simulink model "ControlSystem_new"  (R2019a)
settings: Solver=VariableStepAuto  StartTime=0.0  StopTime=50  RelTol=1e-3
model workspace (MAT data in the model file):
  a_1 = 0
  a_2 = 0
  delta = 0.001
values from neighbouring files (symbols this model uses):
  A = [0 0 0 0 1 0 0 0 0 0 0 0 ... (64 elements, 8x8)]    [IC_4DOF_new.mat]
  a1_dim = 0.409090909091    [IC_4DOF_new.mat]
  a2_dim = 0.409090909091    [IC_4DOF_new.mat]
  Ax_dim = 0.000833333333333    [IC_4DOF_new.mat]
  delta_dim = 1    [IC_4DOF_new.mat]
  h = 0.0002    [IC_4DOF_new.mat]
  h_dim = 0.00909090909091    [IC_4DOF_new.mat]
  i0_dim = 0.0007    [IC_4DOF_new.mat]
  omega = 1047.1975512    [IC_4DOF_new.mat]
  omega_dim = 0.753327454075    [IC_4DOF_new.mat]
  P2 = 8.714    [IC_4DOF_new.mat]
  p_dim = 0    [IC_4DOF_new.mat]
  Pk = 1000000    [IC_4DOF_new.mat]
  Px_dim = 0    [IC_4DOF_new.mat]
  Sf = 1.2    [IC_4DOF_new.mat]
  Sm = 0.000315532958163    [IC_4DOF_new.mat]
  Zb = [1 0 1 0 0 1 0 1 0 0.409090909091 0 -0.409090909091 ... (16 elements, 4x4)]    [IC_4DOF_new.mat]
  Zb_1 = [0.5 0 0 -1.22222222222 0 0.5 1.22222222222 0 0.5 0 0 1.22222222222 ... (16 elements, 4x4)]    [IC_4DOF_new.mat]
libraries: simulink x25, cstblocks x1, neural x1
settings Model: Creator=Vladimir  LastModifiedBy=first
settings SolverCC: AlgebraicLoopSolver=LineSearch
settings DataIOCC: ReturnWorkspaceOutputs=off
settings DebuggingCC: ArithmeticOperatorsInVariantConditions=warning

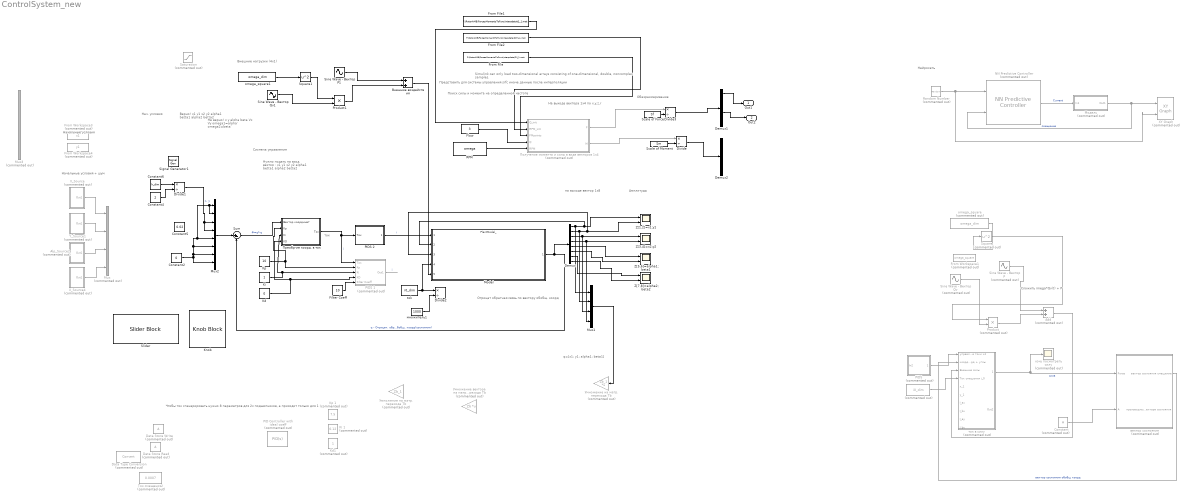
== system ControlSystem_new ==
  note: Представить для системы управления srfc иначе данные после интерполяции
  note: Simulink can only load two-dimensional arrays consisting of one-dimensional, double, noncomplex samples.
  note: Обезразмеривание
  note: На выходе вектора 1х4 по x,y,z,r
  note: Поиск силы и момента на определенной частоте
  note: Не верно!
      | x
      | y
      | alpha
      | beta
      | Vx
      | Vy
      | omega1=alpha'
      | omega2=beta'
  note: Амплитуды
  note: Система управления
  note: на выходе вектор 1x8
  note: Нужно подать на вход вектор :
      | x1
      | y1
      | x2
      | y2
      | alpha1
      | betta1
      | alpha2
      | betta2
  note: q=[x1; y1; alpha1; beta1]
  note: Нач. условия
  note: Чтобы ток сгенерировать нужно 8 параметров для 2х подшипников, а приходит только для 1
  note: Нейросеть
  note: Начальные условия
  note: Отрицат обратная связь по вектору обобщ. коорд
  note: Сложить imega*Qv(t) + P
  note: Начальные условия + шум
  note: ток
  note: Верно!
      | x1
      | y1
      | x2
      | y2
      | alpha1
      | betta1
      | alpha2
      | betta2
  note: Внешние нагрузки (4x1)
  " " : Constant  Commented=on  Value=i0_dim
  " tok" : Constant  Value=i0_dim
  " Ток смещения2" : Constant  Commented=on  Value=0.0007
  " вектор состояния " : Subsystem  Commented=on
  Add : Sum  Commented=on
  Alp_Source2 : Subsystem  Commented=on
  Constant : Constant  Commented=on  Value=A
  Constant2 : Constant  Value=0
  Constant4 : Constant  Value=2
  Constant5 : Constant  Value=0.02
  Constant6 : Constant  Value=h_dim
  Data Store Read : DataStoreRead  Commented=on
  Data Store Write : DataStoreWrite  Commented=on
  Data Type Conversion : DataTypeConversion  Commented=on
  Demux : Demux  Outputs=8
  Demux1 : Demux
  Demux2 : Demux
  Divide{,1..3} (4 alike) : Product  Inputs=*/
  "Filter Coeff " : Constant  Value=10
  "Flow " : Constant  Value=3
  From Workspace1 : FromWorkspace  Commented=on  VariableName=omega_square  SampleTime=0
  From Workspace3 : FromWorkspace  Commented=on  VariableName=x1  SampleTime=0
  From Workspace4 : FromWorkspace  Commented=on  VariableName=y1  SampleTime=0
  From File : FromFile  FileName=F:\RotorAMB\ForcesMomentsToFunc\interpdata\FM_1.mat  SampleTime=0
  From File1 : FromFile  FileName=F:\RotorAMB\ForcesMomentsToFunc\interpdata\Q_1.mat  SampleTime=0
  From File2 : FromFile  FileName=F:\RotorAMB\ForcesMomentsToFunc\interpdata\RPM_1.mat  SampleTime=0
  Kd : Constant  Value=0
  Kd1 : Constant  Commented=on
  "Ki " : Constant
  Ki 1 : Constant  Commented=on  Value=0.12
  Knob : KnobBlock  ScaleMax=5
  "Kp " : Constant  Value=10
  Kp 1 : Constant  Commented=on  Value=7.5
  Model : ModelReference  ModelNameDialog=PlantModel_.slx  SimulationMode=Normal  ModelReferenceVersion=1.39
  Mux : Mux  Commented=on
  Mux1 : Mux
  Mux2 : Mux  Inputs=8
  Mux3 : Mux  Commented=on
  NN Predictive Controller : neural/Control Systems/NN Predictive Controller  Commented=on  epochs=500  minp=[]  maxp=[]  mint=[]  maxt=[]  Normalize=[]  IW=[]  LW1_2=[]  LW2_1=[]  B1=[]  B2=[]  max_i_int=[]  min_i_int=[]  limit_output=[]  max_output=[]  min_output=[]  Use_Previous_Weights=[]  N2=7  Nu=2  Ts=[]  rho=0.05  alpha=0.001  csrchfun=csrchbac  maxiter=2  S1=[]  Ni=[]  Nj=[]  sim_file=0  trainfun=trainlm  Use_validation=[]  Use_Testing=[]  max_i=[]  min_i=[]  sam_training=[]
      settings: SourceProductName=Deep Learning Toolbox  SourceProductBaseCode=NN
  "PID Controller with ideal coeff " : simulink/Continuous/PID Controller  Commented=on  Controller=PID  Form=Parallel  TimeDomain=Continuous-time  SampleTime=-1  IntegratorMethod=Forward Euler  FilterMethod=Forward Euler  ControllerParametersSource=internal  P=7.5  I=0.12  D=1  UseFilter=on  N=100  TunerSelectOption=Transfer Function Based (PID Tuner App)  InitialConditionSource=internal  InitialConditionForIntegrator=0  InitialConditionForFilter=0  DifferentiatorICPrevScaledInput=0  ExternalReset=none  TrackingMode=off  Kt=1  LimitOutput=off  UpperSaturationLimit=inf  LowerSaturationLimit=-inf  LinearizeAsGain=on  AntiWindupMode=none  Kb=1  POutMin=[]  POutMax=[]  IOutMin=[]  IOutMax=[]  DOutMin=[]  DOutMax=[]  NOutMin=[]  NOutMax=[]  SumOutMin=[]  SumOutMax=[]  SaturationOutMin=[]  SaturationOutMax=[]  PParamMin=[]  PParamMax=[]  IParamMin=[]  IParamMax=[]  DParamMin=[]  DParamMax=[]  NParamMin=[]  NParamMax=[]  KbParamMin=[]  KbParamMax=[]  KtParamMin=[]  KtParamMax=[]  KbOutMin=[]  KbOutMax=[]  KtOutMin=[]  KtOutMax=[]  IntegratorOutMin=[]  IntegratorOutMax=[]  FilterOutMin=[]  FilterOutMax=[]  SumI1OutMin=[]  SumI1OutMax=[]  SumI2OutMin=[]  SumI2OutMax=[]  SumI3OutMin=[]  SumI3OutMax=[]  SumI4OutMin=[]  SumI4OutMax=[]  SumDOutMin=[]  SumDOutMax=[]  DifferentiatorOutMin=[]  DifferentiatorOutMax=[]  FilterDiffOutCoefMin=[]  FilterDiffOutCoefMax=[]  ReciprocalOutMin=[]  ReciprocalOutMax=[]  SumDenOutMin=[]  SumDenOutMax=[]  SumNumOutMin=[]  SumNumOutMax=[]  DivideOutMin=[]  DivideOutMax=[]  IntegratorContinuousStateAttributes=''  IntegratorStateMustResolveToSignalObject=off  IntegratorRTWStateStorageClass=Auto  FilterContinuousStateAttributes=''  FilterStateMustResolveToSignalObject=off  FilterRTWStateStorageClass=Auto  ParallelPVariant=InternalParameters  IdealPVariant=Disabled  IVariant=InternalParameters  DVariant=InternalParameters  IntegratorVariant=Continuous  SatVariant=Disabled  AWVariant=Passthrough  PCopyVariant=Disabled  TRVariant=Disabled  FdbkBlocksVariant=Forward  IdealPFdbkVariant=Disabled  SatFdbkVariant=Disabled  DerivativeFilterVariant=ContFilter  NVariant=InternalParameters  NCopyVariant=Disabled  FilterICVariant=InternalICsFilter  IntegratorICVariant=InternalICs  ExternalResetVariant=Disabled  TRSumVariant=Passthrough  SumFdbkVariant=Disabled  SumVariant=Sum_PID
  "PIDS " : Subsystem  Commented=on
  PIDS 1 : Subsystem  Commented=on
  PIDS 2 : Subsystem
  Product : Product  Commented=on
  Product1 : Product
  "RPM " : Constant  Value=omega
  Random Number : RandomNumber  Commented=on  SampleTime=0.1
  Saturation : Saturate  Commented=on  UpperLimit=0.005  LowerLimit=-0.005
  "Scale of Force " : Constant  Value=Sf
  "Scale of Moment " : Constant  Value=Sm
  Signal Generator1 : SignalGenerator  Amplitude=h/2  Units=rad/sec
  Sine Wave - Вектор P : Sin  Commented=on  Amplitude=Ax_dim  Bias=Px_dim  Frequency=p_dim  SampleTime=1
  Sine Wave - Вектор P1 : Sin  Amplitude=Ax_dim  Bias=Px_dim  Frequency=p_dim  SampleTime=1
  Sine Wave - Вектор Qv : Sin  Commented=on  Amplitude=Ax_dim  Bias=Px_dim  Frequency=p_dim  SampleTime=1
  Sine Wave - Вектор Qv1 : Sin  Amplitude=Ax_dim  Bias=Px_dim  Frequency=p_dim  SampleTime=1
  Slider : SliderBlock  ScaleMin=0.01
  Square : Math  Commented=on  Operator=square  SaturateOnIntegerOverflow=on
  Square1 : Math  Operator=square  SaturateOnIntegerOverflow=on
  Sum : Sum  Inputs=|+-
  XY Graph : simulink/Sinks/XY Graph  Commented=on  xmin=-1  xmax=1  ymin=-1  ymax=1  st=-1
  X_Source : Subsystem  Commented=on
  X_Source4 : Subsystem  Commented=on
  Y_Source1 : Subsystem  Commented=on
  "Z[1,2]=x1;y1 " : Scope  NumInputPorts=2
  Z[3,4]=x2;y2 : Scope  NumInputPorts=2
  Z[5,6]=alpha1; beta1 : Scope  NumInputPorts=2
  Z[7,8]=alpha2; beta2 : Scope  NumInputPorts=2
  omega_square : Constant  Commented=on  Value=omega_dim
  omega_square1 : Constant  Value=omega_dim
  Внешние воздействия : Sum
  "Модель " : Subsystem  Commented=on
  Получение момента и силы в виде векторов 1x4 : MATLAB Function  Commented=on  TreatAsAtomicUnit=on
  "Преобр-ие коорд. в ток " : Subsystem
  "Умножение вектора на матр. перехода Tb " : Gain  Commented=on  Gain=Zb  Multiplication=Matrix(K*u) (u vector)
  Умножение на матр. перехода Tb : Gain  Commented=on  Gain=Zb_1  Multiplication=Matrix(K*u)
  "Умножение на матр. перехода Tb " : Gain  Commented=on  Gain=Zb_1
  множитель1 : Constant  Value=1000
  "ток в силу " : Subsystem  Commented=on
  хочу посмотреть силу : Scope  Commented=on
  Out1 : Outport
  Out2 : Outport  Port=2
  wires:
  X_Source/1(Out1) -> Mux/1
  Y_Source1/1(Out1) -> Mux/2
  Alp_Source2/1(Out1) -> Mux/3
  X_Source4/1(Out1) -> Mux/4
  " вектор состояния "/1(вектор состояния смещение) -> "ток в силу "/2(координаты на предидущий такт коорд + углы)  "вектор состояния обобщ коорд"
  "ток в силу "/1(" ") -> хочу посмотреть силу/1, " вектор состояния "/1(Force)  "сила"
  Demux/1 -> "Z[1,2]=x1;y1 "/1, Model/2, Mux1/1
  Demux/2 -> Mux1/2, "Z[1,2]=x1;y1 "/2, Model/3
  Demux/3 -> Mux1/3, Z[3,4]=x2;y2/1
  Demux/4 -> Z[3,4]=x2;y2/2, Mux1/4
  Add/1 -> "ток в силу "/3(Внешние силы)
  Sine Wave - Вектор P/1 -> Add/1
  "PIDS "/1("  ") -> "ток в силу "/1(управляющие токи x4)
  Sine Wave - Вектор Qv/1 -> Product/2
  Product/1 -> Add/2
  " "/1 -> "ток в силу "/4(Ток смещения i_0)
  Constant/1 -> " вектор состояния "/2("A ")
  omega_square/1 -> Square/1
  Square/1 -> Product/1
  Sum/1 -> "Преобр-ие коорд. в ток "/1(Вектор координат)  "Ф=q*-q"
  Random Number/1 -> XY Graph/2, NN Predictive Controller/1
  NN Predictive Controller/1 -> "Модель "/1(In1)  "Current"
  "Модель "/1(Out1) -> NN Predictive Controller/2, XY Graph/1  "смещение"
  Model/1 -> Sum/2, Demux/1  "q - Отрицат. обрат. связь по вектору обобщ. коорд(состояния)"
  Constant2/1 -> Mux2/8, Mux2/6, Mux2/2, Mux2/1, Mux2/5, Mux2/7
  Mux2/1 -> Sum/1
  Constant4/1 -> Divide1/2
  "Kp "/1 -> "Преобр-ие коорд. в ток "/2(Kp), PIDS 1/2(Kp)
  "Ki "/1 -> PIDS 1/3(Ki), "Преобр-ие коорд. в ток "/3(Ki)
  Kd/1 -> PIDS 1/4("KD "), "Преобр-ие коорд. в ток "/4("KD ")
  "Filter Coeff "/1 -> PIDS 1/5(Filter Coeff)
  Constant6/1 -> Divide1/1
  " tok"/1 -> Divide2/1, Model/4
  множитель1/1 -> Divide2/2
  "Преобр-ие коорд. в ток "/1(Ток) -> PIDS 2/1(Ток), PIDS 1/1(Ток)  "i"
  PIDS 2/1("  ") -> Model/1  "i"
  Demux/5 -> Z[5,6]=alpha1; beta1/1
  Demux/6 -> Z[5,6]=alpha1; beta1/2
  Demux/7 -> Z[7,8]=alpha2; beta2/1
  Demux/8 -> Z[7,8]=alpha2; beta2/2
  Mux1/1 -> Умножение на матр. перехода Tb/1
  Divide1/1 -> Mux2/4, Mux2/3  "x, y"
  PIDS 1/1(Out1) -> ?  "i"
  omega_square1/1 -> Square1/1
  Sine Wave - Вектор Qv1/1 -> Product1/2
  Product1/1 -> Внешние воздействия/2
  Sine Wave - Вектор P1/1 -> Внешние воздействия/1
  Square1/1 -> Product1/1
  Внешние воздействия/1 -> Model/5
  Получение момента и силы в виде векторов 1x4/1(F) -> Divide3/1
  Получение момента и силы в виде векторов 1x4/2(M) -> Divide/1
  "Scale of Moment "/1 -> Divide/2
  "Scale of Force "/1 -> Divide3/2
  Divide3/1 -> Demux1/1
  Divide/1 -> Demux2/1
  Demux1/3 -> Out2/1
  Demux1/1 -> Out1/1
  "RPM "/1 -> Получение момента и силы в виде векторов 1x4/5(RPM)
  "Flow "/1 -> Получение момента и силы в виде векторов 1x4/4(Q)
  From File/1 -> Получение момента и силы в виде векторов 1x4/3(FMpoints)
  From File2/1 -> Получение момента и силы в виде векторов 1x4/2(RPM_init)
  From File1/1 -> Получение момента и силы в виде векторов 1x4/1(Q_init)
  ? -> ?

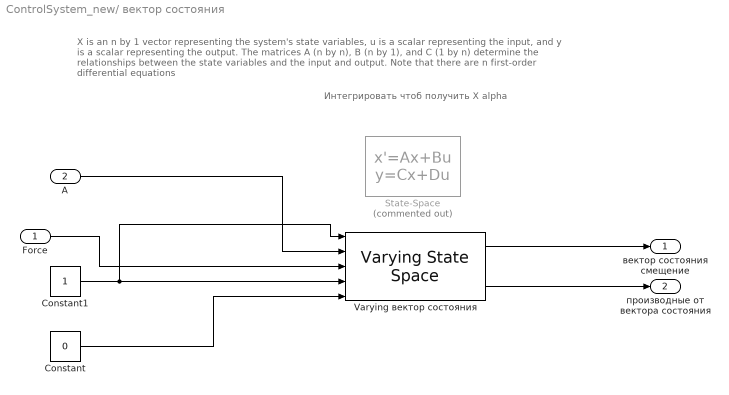
== system ControlSystem_new/ вектор состояния  ==
  note: X is an n by 1 vector representing the system's state variables, u is a scalar representing the input, and y is a scalar representing the output.
      |  The matrices A (n by n), B (n by 1), and C (1 by n) determine the relationships between the state variables and the input and output.
      | Note that there are n first-order differential equations
  note: Интегрировать чтоб получить X alpha
  Force : Inport
  "A " : Inport  Port=2
  Constant : Constant  Value=0
  Constant1 : Constant
  State-Space : StateSpace  Commented=on  InitialCondition=0
  Varying вектор состояния : cstblocks/Linear Parameter Varying/Varying State Space  x0=0  xNames=''  OutputX=on  OutputDX=on
      settings: SourceProductName=Control System Toolbox
  вектор состояния смещение : Outport
  производные от вектора состояния : Outport  Port=2
  wires:
  Force/1 -> Varying вектор состояния/3
  "A "/1 -> Varying вектор состояния/2
  Varying вектор состояния/3 -> производные от вектора состояния/1
  Constant/1 -> Varying вектор состояния/5
  Constant1/1 -> Varying вектор состояния/4, Varying вектор состояния/1
  Varying вектор состояния/1 -> вектор состояния смещение/1

== system ControlSystem_new/Alp_Source2 ==
  note: Tok Here
  note: dtrnjh 4[
  Band-Limited White Noise : simulink/Sources/Band-Limited White Noise  Cov=[0.1]  Ts=0.1  seed=[23341]
  Gain : Gain
  Gain1 : Gain
  Sine Wave : Sin  SampleTime=0
  Step : Step  SampleTime=0
  Sum : Sum  Inputs=|+++
  Out1 : Outport
  wires:
  Gain1/1 -> Sum/3
  Band-Limited White Noise/1 -> Gain/1
  Sine Wave/1 -> Gain1/1
  Step/1 -> Sum/1
  Gain/1 -> Sum/2
  Sum/1 -> Out1/1

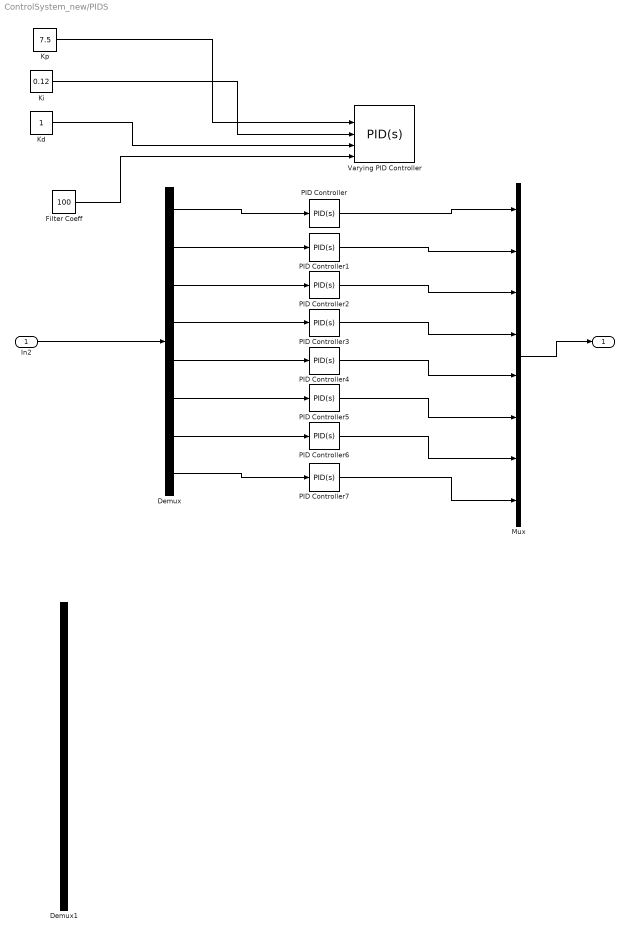
== system ControlSystem_new/PIDS  ==
  In2 : Inport
  Demux : Demux  Outputs=8
  Demux1 : Demux  Outputs=8
  "Filter Coeff " : Constant  Value=100
  Kd : Constant
  "Ki " : Constant  Value=0.12
  "Kp " : Constant  Value=7.5
  Mux : Mux  Inputs=8
  PID Controller{,1..7} (8 alike) : simulink/Continuous/PID Controller  Controller=PID  Form=Parallel  TimeDomain=Continuous-time  SampleTime=-1  IntegratorMethod=Forward Euler  FilterMethod=Forward Euler  ControllerParametersSource=internal  P=1  I=1  D=0  UseFilter=on  N=100  TunerSelectOption=Transfer Function Based (PID Tuner App)  InitialConditionSource=internal  InitialConditionForIntegrator=0  InitialConditionForFilter=0  DifferentiatorICPrevScaledInput=0  ExternalReset=none  TrackingMode=off  Kt=1  LimitOutput=off  UpperSaturationLimit=inf  LowerSaturationLimit=-inf  LinearizeAsGain=on  AntiWindupMode=none  Kb=1  POutMin=[]  POutMax=[]  IOutMin=[]  IOutMax=[]  DOutMin=[]  DOutMax=[]  NOutMin=[]  NOutMax=[]  SumOutMin=[]  SumOutMax=[]  SaturationOutMin=[]  SaturationOutMax=[]  PParamMin=[]  PParamMax=[]  IParamMin=[]  IParamMax=[]  DParamMin=[]  DParamMax=[]  NParamMin=[]  NParamMax=[]  KbParamMin=[]  KbParamMax=[]  KtParamMin=[]  KtParamMax=[]  KbOutMin=[]  KbOutMax=[]  KtOutMin=[]  KtOutMax=[]  IntegratorOutMin=[]  IntegratorOutMax=[]  FilterOutMin=[]  FilterOutMax=[]  SumI1OutMin=[]  SumI1OutMax=[]  SumI2OutMin=[]  SumI2OutMax=[]  SumI3OutMin=[]  SumI3OutMax=[]  SumI4OutMin=[]  SumI4OutMax=[]  SumDOutMin=[]  SumDOutMax=[]  DifferentiatorOutMin=[]  DifferentiatorOutMax=[]  FilterDiffOutCoefMin=[]  FilterDiffOutCoefMax=[]  ReciprocalOutMin=[]  ReciprocalOutMax=[]  SumDenOutMin=[]  SumDenOutMax=[]  SumNumOutMin=[]  SumNumOutMax=[]  DivideOutMin=[]  DivideOutMax=[]  IntegratorContinuousStateAttributes=''  IntegratorStateMustResolveToSignalObject=off  IntegratorRTWStateStorageClass=Auto  FilterContinuousStateAttributes=''  FilterStateMustResolveToSignalObject=off  FilterRTWStateStorageClass=Auto  ParallelPVariant=InternalParameters  IdealPVariant=Disabled  IVariant=InternalParameters  DVariant=InternalParameters  IntegratorVariant=Continuous  SatVariant=Disabled  AWVariant=Passthrough  PCopyVariant=Disabled  TRVariant=Disabled  FdbkBlocksVariant=Forward  IdealPFdbkVariant=Disabled  SatFdbkVariant=Disabled  DerivativeFilterVariant=ContFilter  NVariant=InternalParameters  NCopyVariant=Disabled  FilterICVariant=InternalICsFilter  IntegratorICVariant=InternalICs  ExternalResetVariant=Disabled  TRSumVariant=Passthrough  SumFdbkVariant=Disabled  SumVariant=Sum_PID
  Varying PID Controller : simulink/Continuous/PID Controller  Controller=PID  Form=Parallel  TimeDomain=Continuous-time  SampleTime=-1  IntegratorMethod=Forward Euler  FilterMethod=Forward Euler  ControllerParametersSource=external  P=1  I=1  D=0  UseFilter=on  N=100  TunerSelectOption=Transfer Function Based (PID Tuner App)  InitialConditionSource=internal  InitialConditionForIntegrator=0  InitialConditionForFilter=0  DifferentiatorICPrevScaledInput=0  ExternalReset=none  TrackingMode=off  Kt=1  LimitOutput=off  UpperSaturationLimit=inf  LowerSaturationLimit=-inf  LinearizeAsGain=on  AntiWindupMode=none  Kb=1  POutMin=[]  POutMax=[]  IOutMin=[]  IOutMax=[]  DOutMin=[]  DOutMax=[]  NOutMin=[]  NOutMax=[]  SumOutMin=[]  SumOutMax=[]  SaturationOutMin=[]  SaturationOutMax=[]  PParamMin=[]  PParamMax=[]  IParamMin=[]  IParamMax=[]  DParamMin=[]  DParamMax=[]  NParamMin=[]  NParamMax=[]  KbParamMin=[]  KbParamMax=[]  KtParamMin=[]  KtParamMax=[]  KbOutMin=[]  KbOutMax=[]  KtOutMin=[]  KtOutMax=[]  IntegratorOutMin=[]  IntegratorOutMax=[]  FilterOutMin=[]  FilterOutMax=[]  SumI1OutMin=[]  SumI1OutMax=[]  SumI2OutMin=[]  SumI2OutMax=[]  SumI3OutMin=[]  SumI3OutMax=[]  SumI4OutMin=[]  SumI4OutMax=[]  SumDOutMin=[]  SumDOutMax=[]  DifferentiatorOutMin=[]  DifferentiatorOutMax=[]  FilterDiffOutCoefMin=[]  FilterDiffOutCoefMax=[]  ReciprocalOutMin=[]  ReciprocalOutMax=[]  SumDenOutMin=[]  SumDenOutMax=[]  SumNumOutMin=[]  SumNumOutMax=[]  DivideOutMin=[]  DivideOutMax=[]  IntegratorContinuousStateAttributes=''  IntegratorStateMustResolveToSignalObject=off  IntegratorRTWStateStorageClass=Auto  FilterContinuousStateAttributes=''  FilterStateMustResolveToSignalObject=off  FilterRTWStateStorageClass=Auto  ParallelPVariant=ExternalParameters  IdealPVariant=Disabled  IVariant=ExternalParameters  DVariant=ExternalParameters  IntegratorVariant=Continuous  SatVariant=Disabled  AWVariant=Passthrough  PCopyVariant=Disabled  TRVariant=Disabled  FdbkBlocksVariant=Forward  IdealPFdbkVariant=Disabled  SatFdbkVariant=Disabled  DerivativeFilterVariant=ContFilter  NVariant=ExternalParameters  NCopyVariant=Disabled  FilterICVariant=InternalICsFilter  IntegratorICVariant=InternalICs  ExternalResetVariant=Disabled  TRSumVariant=Passthrough  SumFdbkVariant=Disabled  SumVariant=Sum_PID
  "  " : Outport
  wires:
  Demux/1 -> PID Controller/1
  Demux/2 -> PID Controller1/1
  Demux/3 -> PID Controller2/1
  Demux/4 -> PID Controller3/1
  In2/1 -> Demux/1
  Demux/5 -> PID Controller4/1
  Demux/6 -> PID Controller5/1
  Demux/7 -> PID Controller6/1
  Demux/8 -> PID Controller7/1
  PID Controller/1 -> Mux/1
  PID Controller1/1 -> Mux/2
  PID Controller2/1 -> Mux/3
  PID Controller3/1 -> Mux/4
  PID Controller4/1 -> Mux/5
  PID Controller5/1 -> Mux/6
  PID Controller6/1 -> Mux/7
  PID Controller7/1 -> Mux/8
  Mux/1 -> "  "/1
  "Kp "/1 -> Varying PID Controller/2
  "Filter Coeff "/1 -> Varying PID Controller/5
  "Ki "/1 -> Varying PID Controller/3
  Kd/1 -> Varying PID Controller/4

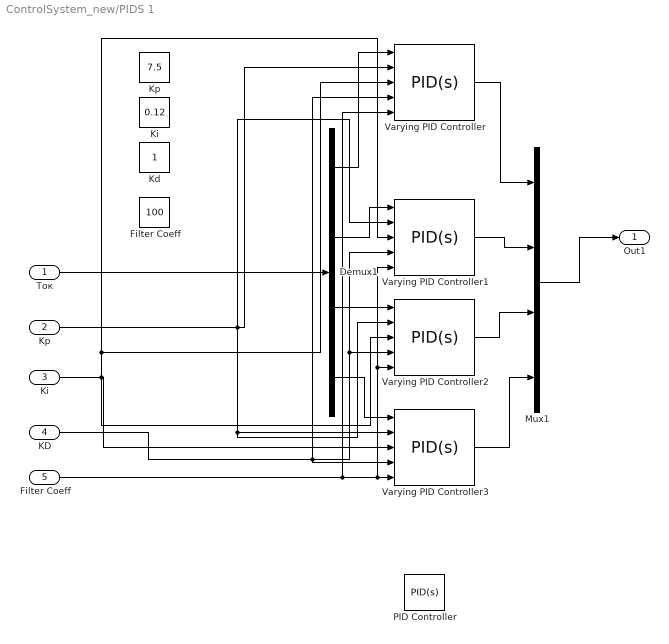
== system ControlSystem_new/PIDS 1 ==
  Ток : Inport
  Kp : Inport  Port=2
  Ki : Inport  Port=3
  "KD " : Inport  Port=4
  Filter Coeff : Inport  Port=5
  Demux1 : Demux
  "Filter Coeff " : Constant  Value=100
  Kd : Constant
  "Ki " : Constant  Value=0.12
  "Kp " : Constant  Value=7.5
  Mux1 : Mux
  PID Controller : simulink/Continuous/PID Controller  Controller=PID  Form=Parallel  TimeDomain=Continuous-time  SampleTime=-1  IntegratorMethod=Forward Euler  FilterMethod=Forward Euler  ControllerParametersSource=internal  P=1  I=1  D=0  UseFilter=on  N=100  TunerSelectOption=Transfer Function Based (PID Tuner App)  InitialConditionSource=internal  InitialConditionForIntegrator=0  InitialConditionForFilter=0  DifferentiatorICPrevScaledInput=0  ExternalReset=none  TrackingMode=off  Kt=1  LimitOutput=off  UpperSaturationLimit=inf  LowerSaturationLimit=-inf  LinearizeAsGain=on  AntiWindupMode=none  Kb=1  POutMin=[]  POutMax=[]  IOutMin=[]  IOutMax=[]  DOutMin=[]  DOutMax=[]  NOutMin=[]  NOutMax=[]  SumOutMin=[]  SumOutMax=[]  SaturationOutMin=[]  SaturationOutMax=[]  PParamMin=[]  PParamMax=[]  IParamMin=[]  IParamMax=[]  DParamMin=[]  DParamMax=[]  NParamMin=[]  NParamMax=[]  KbParamMin=[]  KbParamMax=[]  KtParamMin=[]  KtParamMax=[]  KbOutMin=[]  KbOutMax=[]  KtOutMin=[]  KtOutMax=[]  IntegratorOutMin=[]  IntegratorOutMax=[]  FilterOutMin=[]  FilterOutMax=[]  SumI1OutMin=[]  SumI1OutMax=[]  SumI2OutMin=[]  SumI2OutMax=[]  SumI3OutMin=[]  SumI3OutMax=[]  SumI4OutMin=[]  SumI4OutMax=[]  SumDOutMin=[]  SumDOutMax=[]  DifferentiatorOutMin=[]  DifferentiatorOutMax=[]  FilterDiffOutCoefMin=[]  FilterDiffOutCoefMax=[]  ReciprocalOutMin=[]  ReciprocalOutMax=[]  SumDenOutMin=[]  SumDenOutMax=[]  SumNumOutMin=[]  SumNumOutMax=[]  DivideOutMin=[]  DivideOutMax=[]  IntegratorContinuousStateAttributes=''  IntegratorStateMustResolveToSignalObject=off  IntegratorRTWStateStorageClass=Auto  FilterContinuousStateAttributes=''  FilterStateMustResolveToSignalObject=off  FilterRTWStateStorageClass=Auto  ParallelPVariant=InternalParameters  IdealPVariant=Disabled  IVariant=InternalParameters  DVariant=InternalParameters  IntegratorVariant=Continuous  SatVariant=Disabled  AWVariant=Passthrough  PCopyVariant=Disabled  TRVariant=Disabled  FdbkBlocksVariant=Forward  IdealPFdbkVariant=Disabled  SatFdbkVariant=Disabled  DerivativeFilterVariant=ContFilter  NVariant=InternalParameters  NCopyVariant=Disabled  FilterICVariant=InternalICsFilter  IntegratorICVariant=InternalICs  ExternalResetVariant=Disabled  TRSumVariant=Passthrough  SumFdbkVariant=Disabled  SumVariant=Sum_PID
  Varying PID Controller{,1..3} (4 alike) : simulink/Continuous/PID Controller  Controller=PID  Form=Parallel  TimeDomain=Continuous-time  SampleTime=-1  IntegratorMethod=Forward Euler  FilterMethod=Forward Euler  ControllerParametersSource=external  P=1  I=1  D=0  UseFilter=on  N=100  TunerSelectOption=Transfer Function Based (PID Tuner App)  InitialConditionSource=internal  InitialConditionForIntegrator=0  InitialConditionForFilter=0  DifferentiatorICPrevScaledInput=0  ExternalReset=none  TrackingMode=off  Kt=1  LimitOutput=off  UpperSaturationLimit=inf  LowerSaturationLimit=-inf  LinearizeAsGain=on  AntiWindupMode=none  Kb=1  POutMin=[]  POutMax=[]  IOutMin=[]  IOutMax=[]  DOutMin=[]  DOutMax=[]  NOutMin=[]  NOutMax=[]  SumOutMin=[]  SumOutMax=[]  SaturationOutMin=[]  SaturationOutMax=[]  PParamMin=[]  PParamMax=[]  IParamMin=[]  IParamMax=[]  DParamMin=[]  DParamMax=[]  NParamMin=[]  NParamMax=[]  KbParamMin=[]  KbParamMax=[]  KtParamMin=[]  KtParamMax=[]  KbOutMin=[]  KbOutMax=[]  KtOutMin=[]  KtOutMax=[]  IntegratorOutMin=[]  IntegratorOutMax=[]  FilterOutMin=[]  FilterOutMax=[]  SumI1OutMin=[]  SumI1OutMax=[]  SumI2OutMin=[]  SumI2OutMax=[]  SumI3OutMin=[]  SumI3OutMax=[]  SumI4OutMin=[]  SumI4OutMax=[]  SumDOutMin=[]  SumDOutMax=[]  DifferentiatorOutMin=[]  DifferentiatorOutMax=[]  FilterDiffOutCoefMin=[]  FilterDiffOutCoefMax=[]  ReciprocalOutMin=[]  ReciprocalOutMax=[]  SumDenOutMin=[]  SumDenOutMax=[]  SumNumOutMin=[]  SumNumOutMax=[]  DivideOutMin=[]  DivideOutMax=[]  IntegratorContinuousStateAttributes=''  IntegratorStateMustResolveToSignalObject=off  IntegratorRTWStateStorageClass=Auto  FilterContinuousStateAttributes=''  FilterStateMustResolveToSignalObject=off  FilterRTWStateStorageClass=Auto  ParallelPVariant=ExternalParameters  IdealPVariant=Disabled  IVariant=ExternalParameters  DVariant=ExternalParameters  IntegratorVariant=Continuous  SatVariant=Disabled  AWVariant=Passthrough  PCopyVariant=Disabled  TRVariant=Disabled  FdbkBlocksVariant=Forward  IdealPFdbkVariant=Disabled  SatFdbkVariant=Disabled  DerivativeFilterVariant=ContFilter  NVariant=ExternalParameters  NCopyVariant=Disabled  FilterICVariant=InternalICsFilter  IntegratorICVariant=InternalICs  ExternalResetVariant=Disabled  TRSumVariant=Passthrough  SumFdbkVariant=Disabled  SumVariant=Sum_PID
  Out1 : Outport
  wires:
  Ток/1 -> Demux1/1
  Demux1/1 -> Varying PID Controller/1
  Varying PID Controller/1 -> Mux1/1
  Demux1/2 -> Varying PID Controller1/1
  Varying PID Controller1/1 -> Mux1/2
  Demux1/3 -> Varying PID Controller2/1
  Varying PID Controller2/1 -> Mux1/3
  Demux1/4 -> Varying PID Controller3/1
  Varying PID Controller3/1 -> Mux1/4
  Filter Coeff/1 -> Varying PID Controller/5, Varying PID Controller1/5, Varying PID Controller2/5, Varying PID Controller3/5
  "KD "/1 -> Varying PID Controller/4, Varying PID Controller1/4, Varying PID Controller2/4, Varying PID Controller3/4
  Ki/1 -> Varying PID Controller/3, Varying PID Controller1/3, Varying PID Controller2/3, Varying PID Controller3/3
  Kp/1 -> Varying PID Controller3/2, Varying PID Controller2/2, Varying PID Controller1/2, Varying PID Controller/2
  Mux1/1 -> Out1/1

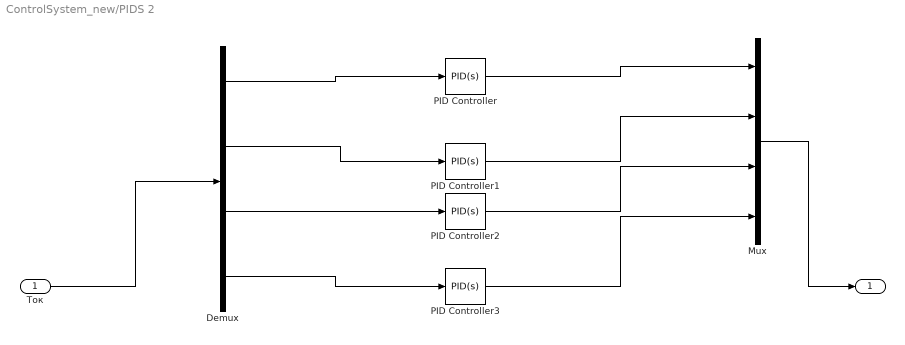
== system ControlSystem_new/PIDS 2 ==
  Ток : Inport
  Demux : Demux
  Mux : Mux
  PID Controller{,1..3} (4 alike) : simulink/Continuous/PID Controller  Controller=PID  Form=Parallel  TimeDomain=Continuous-time  SampleTime=-1  IntegratorMethod=Forward Euler  FilterMethod=Forward Euler  ControllerParametersSource=internal  P=1  I=1  D=1  UseFilter=on  N=100  TunerSelectOption=Transfer Function Based (PID Tuner App)  InitialConditionSource=internal  InitialConditionForIntegrator=0  InitialConditionForFilter=0  DifferentiatorICPrevScaledInput=0  ExternalReset=none  TrackingMode=off  Kt=1  LimitOutput=off  UpperSaturationLimit=inf  LowerSaturationLimit=-inf  LinearizeAsGain=on  AntiWindupMode=none  Kb=1  POutMin=[]  POutMax=[]  IOutMin=[]  IOutMax=[]  DOutMin=[]  DOutMax=[]  NOutMin=[]  NOutMax=[]  SumOutMin=[]  SumOutMax=[]  SaturationOutMin=[]  SaturationOutMax=[]  PParamMin=[]  PParamMax=[]  IParamMin=[]  IParamMax=[]  DParamMin=[]  DParamMax=[]  NParamMin=[]  NParamMax=[]  KbParamMin=[]  KbParamMax=[]  KtParamMin=[]  KtParamMax=[]  KbOutMin=[]  KbOutMax=[]  KtOutMin=[]  KtOutMax=[]  IntegratorOutMin=[]  IntegratorOutMax=[]  FilterOutMin=[]  FilterOutMax=[]  SumI1OutMin=[]  SumI1OutMax=[]  SumI2OutMin=[]  SumI2OutMax=[]  SumI3OutMin=[]  SumI3OutMax=[]  SumI4OutMin=[]  SumI4OutMax=[]  SumDOutMin=[]  SumDOutMax=[]  DifferentiatorOutMin=[]  DifferentiatorOutMax=[]  FilterDiffOutCoefMin=[]  FilterDiffOutCoefMax=[]  ReciprocalOutMin=[]  ReciprocalOutMax=[]  SumDenOutMin=[]  SumDenOutMax=[]  SumNumOutMin=[]  SumNumOutMax=[]  DivideOutMin=[]  DivideOutMax=[]  IntegratorContinuousStateAttributes=''  IntegratorStateMustResolveToSignalObject=off  IntegratorRTWStateStorageClass=Auto  FilterContinuousStateAttributes=''  FilterStateMustResolveToSignalObject=off  FilterRTWStateStorageClass=Auto  ParallelPVariant=InternalParameters  IdealPVariant=Disabled  IVariant=InternalParameters  DVariant=InternalParameters  IntegratorVariant=Continuous  SatVariant=Disabled  AWVariant=Passthrough  PCopyVariant=Disabled  TRVariant=Disabled  FdbkBlocksVariant=Forward  IdealPFdbkVariant=Disabled  SatFdbkVariant=Disabled  DerivativeFilterVariant=ContFilter  NVariant=InternalParameters  NCopyVariant=Disabled  FilterICVariant=InternalICsFilter  IntegratorICVariant=InternalICs  ExternalResetVariant=Disabled  TRSumVariant=Passthrough  SumFdbkVariant=Disabled  SumVariant=Sum_PID
  "  " : Outport
  wires:
  Demux/2 -> PID Controller1/1
  Demux/3 -> PID Controller2/1
  Demux/4 -> PID Controller3/1
  Ток/1 -> Demux/1
  PID Controller1/1 -> Mux/2
  PID Controller2/1 -> Mux/3
  PID Controller3/1 -> Mux/4
  Mux/1 -> "  "/1
  PID Controller/1 -> Mux/1
  Demux/1 -> PID Controller/1

== system ControlSystem_new/X_Source ==
  note: Tok Here
  note: dtrnjh 4[
  Band-Limited White Noise : simulink/Sources/Band-Limited White Noise  Cov=[0.1]  Ts=0.1  seed=[23341]
  Gain : Gain
  Gain1 : Gain
  Sine Wave : Sin  SampleTime=0
  Step : Step  SampleTime=0
  Sum : Sum  Inputs=|+++
  Out1 : Outport
  wires:
  Gain1/1 -> Sum/3
  Band-Limited White Noise/1 -> Gain/1
  Sine Wave/1 -> Gain1/1
  Step/1 -> Sum/1
  Gain/1 -> Sum/2
  Sum/1 -> Out1/1

== system ControlSystem_new/X_Source4 ==
  note: Tok Here
  note: dtrnjh 4[
  Band-Limited White Noise : simulink/Sources/Band-Limited White Noise  Cov=[0.1]  Ts=0.1  seed=[23341]
  Gain : Gain
  Gain1 : Gain
  Sine Wave : Sin  SampleTime=0
  Step : Step  SampleTime=0
  Sum : Sum  Inputs=|+++
  Out1 : Outport
  wires:
  Gain1/1 -> Sum/3
  Band-Limited White Noise/1 -> Gain/1
  Sine Wave/1 -> Gain1/1
  Step/1 -> Sum/1
  Gain/1 -> Sum/2
  Sum/1 -> Out1/1

== system ControlSystem_new/Y_Source1 ==
  note: Tok Here
  note: dtrnjh 4[
  Band-Limited White Noise : simulink/Sources/Band-Limited White Noise  Cov=[0.1]  Ts=0.1  seed=[23341]
  Gain : Gain
  Gain1 : Gain
  Ramp : simulink/Sources/Ramp  slope=1  start=0  InitialOutput=0
  Sine Wave : Sin  SampleTime=0
  Step : Step  SampleTime=0
  Sum : Sum  Inputs=|+++
  Out1 : Outport
  wires:
  Gain1/1 -> Sum/3
  Band-Limited White Noise/1 -> Gain/1
  Sine Wave/1 -> Gain1/1
  Step/1 -> Sum/1
  Gain/1 -> Sum/2
  Sum/1 -> Out1/1
  Ramp/1 -> ?

== system ControlSystem_new/Модель  ==
  In1 : Inport
  Out1 : Outport
  wires:
  In1/1 -> Out1/1

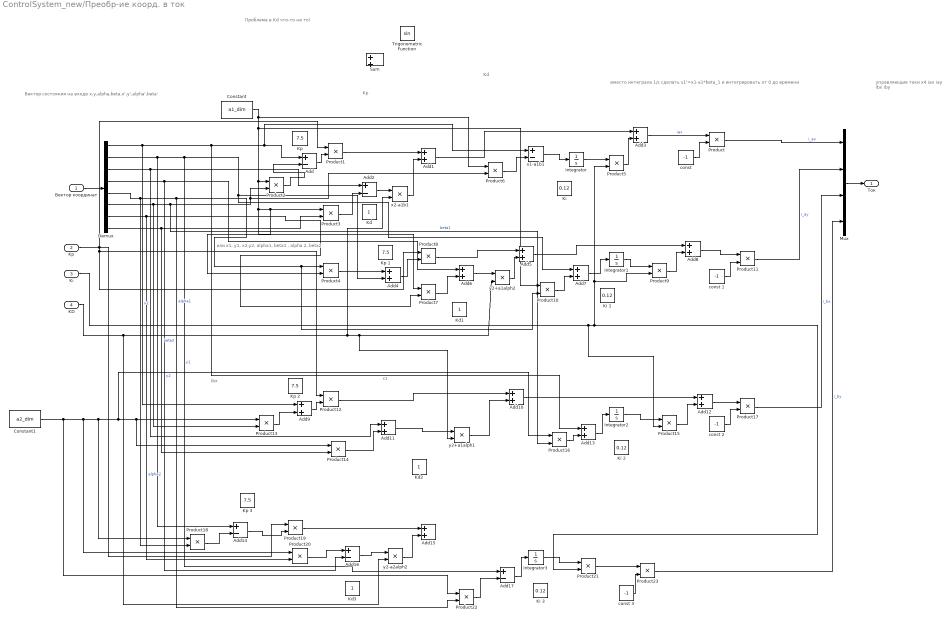
== system ControlSystem_new/Преобр-ие коорд. в ток  ==
  note: Проблема в Kd что-то не то!
  note: Kp
  note: Kd
  note: вместо интеграла 1/s сделать s1'=x1-a1*beta_1 и интегрировать от 0 до времени
  note: Ibx
  note: или x1, y1, x2,y2, alpha1, beta1 , alpha 2, beta2
  note: управляющие токи x4
      | iax iay ibx iby
  note: Вектор состояния на входе x,y,alpha,beta,x',y',alpha',beta'
  Вектор координат : Inport
  Kp : Inport  Port=2
  Ki : Inport  Port=3
  "KD " : Inport  Port=4
  Add{,2,14,16..17} (5 alike) : Sum  Inputs=+-
  Add{1,3..13,15} (13 alike) : Sum
  Constant : Constant  Value=a1_dim
  Constant1 : Constant  Value=a2_dim
  Demux : Demux  Outputs=8
  Integrator : Integrator
  Integrator1 : Integrator
  Integrator2 : Integrator  UpperSaturationLimit=1  LowerSaturationLimit=0.001
  Integrator3 : Integrator
  Kd{,1..3} (4 alike) : Constant
  Ki {,1..3} (4 alike) : Constant  Value=0.12
  Kp {,1..3} (4 alike) : Constant  Value=7.5
  Mux : Mux
  Product{,1..23} (24 alike) : Product
  Sum : Sum  Inputs=|++
  Trigonometric Function : Trigonometry
  const {,1..3} (4 alike) : Constant  Value=-1
  x1-a1b1 : Sum  Inputs=+-
  x2-a1b1 : Product
  y2+a1alph1 : Product
  y2+a1alph2 : Product
  y2-a2alph2 : Product
  Ток : Outport
  wires:
  Mux/1 -> Ток/1
  Вектор координат/1 -> Demux/1
  "const "/1 -> Product/2
  Demux/1 -> Add9/1, x1-a1b1/1, Add/1, Add13/1  "x1"
  Product2/1 -> Add/2
  Add/1 -> Product1/2
  Product1/1 -> Add1/1
  Demux/2 -> Add14/1, Add17/1, Add7/1, Add4/2  "y1"
  Demux/3 -> Add11/1, Add2/1  "x2"
  Demux/4 -> Add16/2, Add6/1  "y2"
  Demux/5 -> Product18/2, Product22/2, Product10/2, Product4/1  "alpha1"
  Demux/6 -> Product13/2, Product16/2, Product6/2, Product2/2  "beta1"
  Demux/7 -> Product20/2, Product7/2  "alpha2"
  Demux/8 -> Product14/2, Product3/2  "beta2"
  Product3/1 -> Add2/2
  Add2/1 -> x2-a1b1/1
  x2-a1b1/1 -> Add1/2
  Product6/1 -> x1-a1b1/2
  Add1/1 -> Add3/1
  x1-a1b1/1 -> Integrator/1
  Integrator/1 -> Product5/1
  Product5/1 -> Add3/2
  Add3/1 -> Product/1  "iax"
  Product/1 -> Mux/1  "i_ax"
  Constant/1 -> Product7/1, Product4/2, Product3/1, Product2/1, Product10/1, Product6/1
  Product4/1 -> Add4/1
  Product7/1 -> Add6/2
  Add6/1 -> y2+a1alph2/1
  y2+a1alph2/1 -> Add5/2
  Add4/1 -> Product8/2
  Product8/1 -> Add5/1
  Integrator1/1 -> Product9/1
  Product10/1 -> Add7/2
  Add7/1 -> Integrator1/1
  Product9/1 -> Add8/2
  Add5/1 -> Add8/1
  const 1/1 -> Product11/2
  Add8/1 -> Product11/1
  Product11/1 -> Mux/2  "i_ay"
  Add9/1 -> Product12/2
  Product13/1 -> Add9/2
  Constant1/1 -> Product22/1, Product20/1, Product18/1, Product16/1, Product14/1, Product13/1
  Product12/1 -> Add10/1
  y2+a1alph1/1 -> Add10/2
  Add11/1 -> y2+a1alph1/1
  Product14/1 -> Add11/2
  Add10/1 -> Add12/1
  Integrator2/1 -> Product15/1
  Product15/1 -> Add12/2
  Product16/1 -> Add13/2
  Add13/1 -> Integrator2/1
  const 2/1 -> Product17/2
  Add12/1 -> Product17/1
  Product17/1 -> Mux/3  "i_bx"
  Product18/1 -> Add14/2
  Add14/1 -> Product19/2
  Product19/1 -> Add15/1
  y2-a2alph2/1 -> Add15/2
  Product20/1 -> Add16/1
  Add16/1 -> y2-a2alph2/1
  Add17/1 -> Integrator3/1
  Integrator3/1 -> Product21/1
  Product22/1 -> Add17/2
  const 3/1 -> Product23/2
  Product21/1 -> Product23/1
  Product23/1 -> Mux/4  "i_by"
  Kp/1 -> Product8/1, Product12/1, Product19/1, Product1/1
  Ki/1 -> Product21/2, Product9/2, Product5/2, Product15/2
  "KD "/1 -> x2-a1b1/2, y2+a1alph1/2, y2+a1alph2/2, y2-a2alph2/2

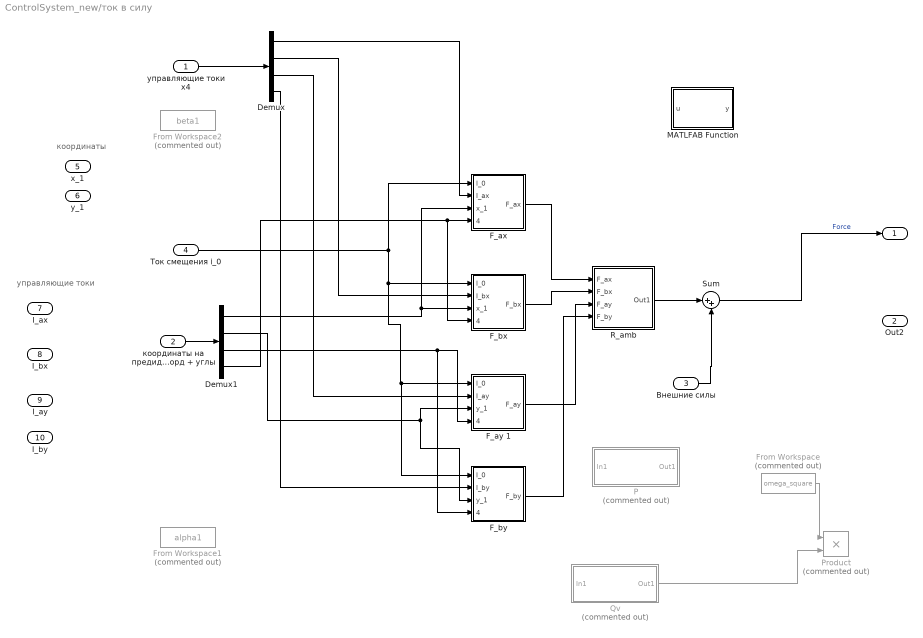
== system ControlSystem_new/ток в силу  ==
  note: координаты
  note: управляющие токи
  управляющие токи x4 : Inport
  координаты на предидущий такт коорд + углы : Inport  Port=2
  Внешние силы : Inport  Port=3
  Ток смещения i_0 : Inport  Port=4
  x_1 : Inport  Port=5
  y_1 : Inport  Port=6
  I_ax : Inport  Port=7
  I_bx : Inport  Port=8
  I_ay : Inport  Port=9
  I_by : Inport  Port=10
  Demux : Demux
  Demux1 : Demux
  F_ax : Subsystem
  F_ay 1 : Subsystem
  F_bx : Subsystem
  F_by : Subsystem
  From Workspace : FromWorkspace  Commented=on  VariableName=omega_square  SampleTime=0
  From Workspace1 : FromWorkspace  Commented=on  VariableName=alpha1  SampleTime=0
  From Workspace2 : FromWorkspace  Commented=on  VariableName=beta1  SampleTime=0
  MATLFAB Function : MATLAB Function  TreatAsAtomicUnit=on
  P : Subsystem  Commented=on
  Product : Product  Commented=on
  Qv : Subsystem  Commented=on
  R_amb : Subsystem
  Sum : Sum  Inputs=|++
  " " : Outport
  Out2 : Outport  Port=2
  wires:
  F_ax/1(F_ax) -> R_amb/1(F_ax)
  F_bx/1(F_bx) -> R_amb/2(F_bx)
  F_ay 1/1(F_ay) -> R_amb/3(F_ay)
  F_by/1(F_by) -> R_amb/4(F_by)
  R_amb/1(Out1) -> Sum/1
  Sum/1 -> " "/1  "Force"
  From Workspace/1 -> Product/1
  Qv/1(Out1) -> Product/2
  Внешние силы/1 -> Sum/2
  Ток смещения i_0/1 -> F_by/1(I_0), F_ay 1/1(I_0), F_bx/1(I_0), F_ax/1(I_0)
  управляющие токи x4/1 -> Demux/1
  Demux/1 -> F_ax/2(I_ax)
  Demux/2 -> F_bx/2(I_bx)
  Demux/3 -> F_ay 1/2(I_ay)
  Demux/4 -> F_by/2(I_by)
  координаты на предидущий такт коорд + углы/1 -> Demux1/1
  Demux1/1 -> F_ax/3(x_1), F_bx/3(x_1)
  Demux1/2 -> F_by/3(y_1), F_ay 1/3(y_1)
  Demux1/3 -> F_by/4(alpha_1), F_ay 1/4(alpha_1)
  Demux1/4 -> F_bx/4(betta_1), F_ax/4(betta_1)

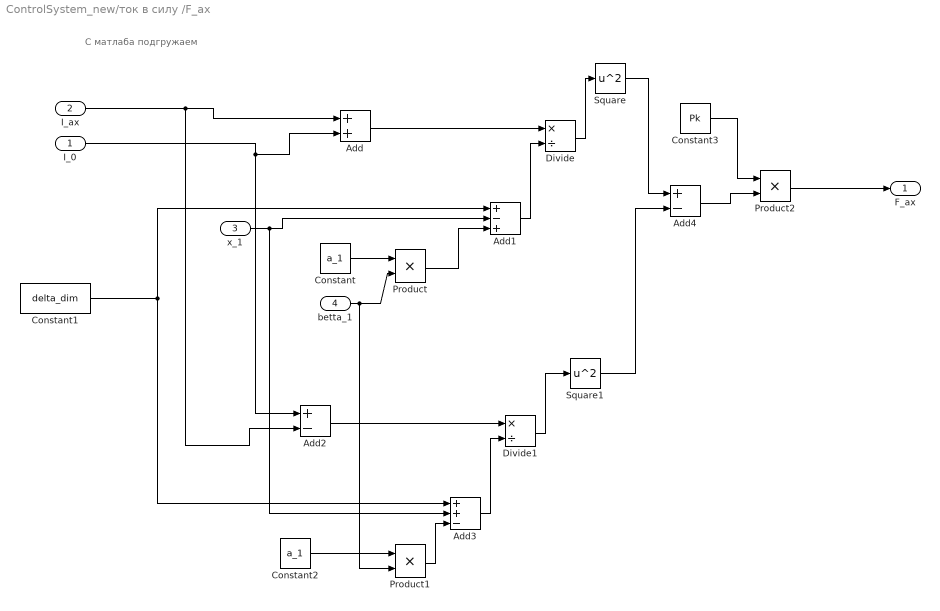
== system ControlSystem_new/ток в силу /F_ax ==
  note: С матлаба подгружаем
  I_0 : Inport
  I_ax : Inport  Port=2
  x_1 : Inport  Port=3
  betta_1 : Inport  Port=4
  Add : Sum
  Add1 : Sum  Inputs=+-+
  Add2 : Sum  Inputs=+-
  Add3 : Sum  Inputs=++-
  Add4 : Sum  Inputs=+-
  Constant : Constant  Value=a_1
  Constant1 : Constant  Value=delta_dim
  Constant2 : Constant  Value=a_1
  Constant3 : Constant  Value=Pk
  Divide : Product  Inputs=*/
  Divide1 : Product  Inputs=*/
  Product : Product
  Product1 : Product
  Product2 : Product
  Square : Math  Operator=square  SaturateOnIntegerOverflow=on
  Square1 : Math  Operator=square  SaturateOnIntegerOverflow=on
  F_ax : Outport
  wires:
  Product2/1 -> F_ax/1
  Constant/1 -> Product/1
  Product/1 -> Add1/3
  Add1/1 -> Divide/2
  Add/1 -> Divide/1
  Divide/1 -> Square/1
  Product1/1 -> Add3/3
  Add2/1 -> Divide1/1
  Constant2/1 -> Product1/1
  I_ax/1 -> Add2/2, Add/1
  Add3/1 -> Divide1/2
  x_1/1 -> Add1/2, Add3/2
  Divide1/1 -> Square1/1
  I_0/1 -> Add/2, Add2/1
  betta_1/1 -> Product/2, Product1/2
  Square/1 -> Add4/1
  Square1/1 -> Add4/2
  Constant3/1 -> Product2/1
  Add4/1 -> Product2/2
  Constant1/1 -> Add1/1, Add3/1

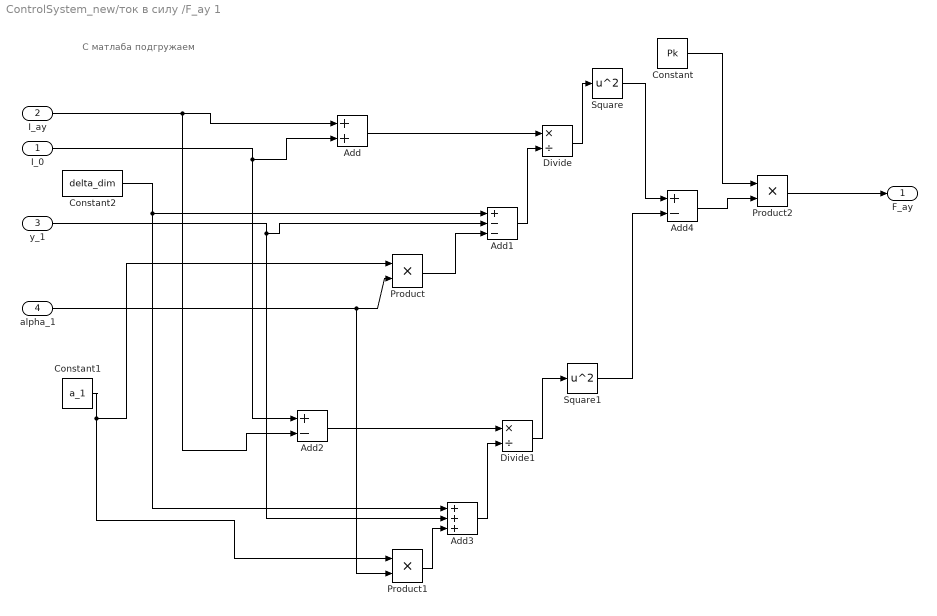
== system ControlSystem_new/ток в силу /F_ay 1 ==
  note: С матлаба подгружаем
  I_0 : Inport
  I_ay : Inport  Port=2
  y_1 : Inport  Port=3
  alpha_1 : Inport  Port=4
  Add : Sum
  Add1 : Sum  Inputs=+--
  Add2 : Sum  Inputs=+-
  Add3 : Sum  Inputs=+++
  Add4 : Sum  Inputs=+-
  Constant : Constant  Value=Pk
  Constant1 : Constant  Value=a_1
  Constant2 : Constant  Value=delta_dim
  Divide : Product  Inputs=*/
  Divide1 : Product  Inputs=*/
  Product : Product
  Product1 : Product
  Product2 : Product
  Square : Math  Operator=square  SaturateOnIntegerOverflow=on
  Square1 : Math  Operator=square  SaturateOnIntegerOverflow=on
  F_ay : Outport
  wires:
  Product2/1 -> F_ay/1
  Product/1 -> Add1/3
  Add1/1 -> Divide/2
  Add/1 -> Divide/1
  Divide/1 -> Square/1
  Product1/1 -> Add3/3
  Add2/1 -> Divide1/1
  Constant1/1 -> Product1/1, Product/1
  I_ay/1 -> Add2/2, Add/1
  Add3/1 -> Divide1/2
  y_1/1 -> Add1/2, Add3/2
  Divide1/1 -> Square1/1
  I_0/1 -> Add/2, Add2/1
  alpha_1/1 -> Product/2, Product1/2
  Square/1 -> Add4/1
  Square1/1 -> Add4/2
  Constant/1 -> Product2/1
  Add4/1 -> Product2/2
  Constant2/1 -> Add3/1, Add1/1

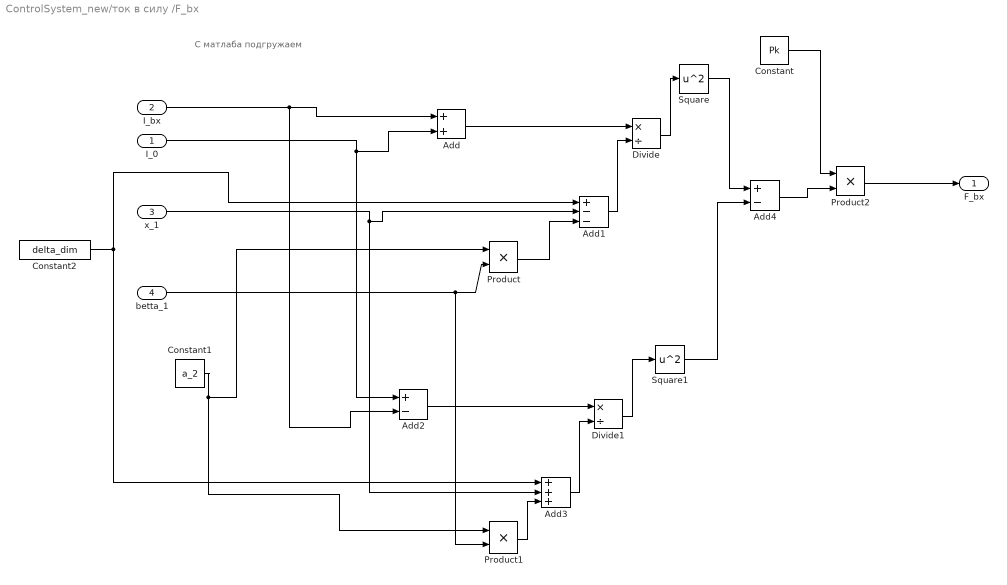
== system ControlSystem_new/ток в силу /F_bx ==
  note: С матлаба подгружаем
  I_0 : Inport
  I_bx : Inport  Port=2
  x_1 : Inport  Port=3
  betta_1 : Inport  Port=4
  Add : Sum
  Add1 : Sum  Inputs=+--
  Add2 : Sum  Inputs=+-
  Add3 : Sum  Inputs=+++
  Add4 : Sum  Inputs=+-
  Constant : Constant  Value=Pk
  Constant1 : Constant  Value=a_2
  Constant2 : Constant  Value=delta_dim
  Divide : Product  Inputs=*/
  Divide1 : Product  Inputs=*/
  Product : Product
  Product1 : Product
  Product2 : Product
  Square : Math  Operator=square  SaturateOnIntegerOverflow=on
  Square1 : Math  Operator=square  SaturateOnIntegerOverflow=on
  F_bx : Outport
  wires:
  Product2/1 -> F_bx/1
  Product/1 -> Add1/3
  Add1/1 -> Divide/2
  Add/1 -> Divide/1
  Divide/1 -> Square/1
  Product1/1 -> Add3/3
  Add2/1 -> Divide1/1
  Constant1/1 -> Product1/1, Product/1
  I_bx/1 -> Add2/2, Add/1
  Add3/1 -> Divide1/2
  x_1/1 -> Add1/2, Add3/2
  Divide1/1 -> Square1/1
  I_0/1 -> Add/2, Add2/1
  betta_1/1 -> Product/2, Product1/2
  Square/1 -> Add4/1
  Square1/1 -> Add4/2
  Constant/1 -> Product2/1
  Add4/1 -> Product2/2
  Constant2/1 -> Add1/1, Add3/1

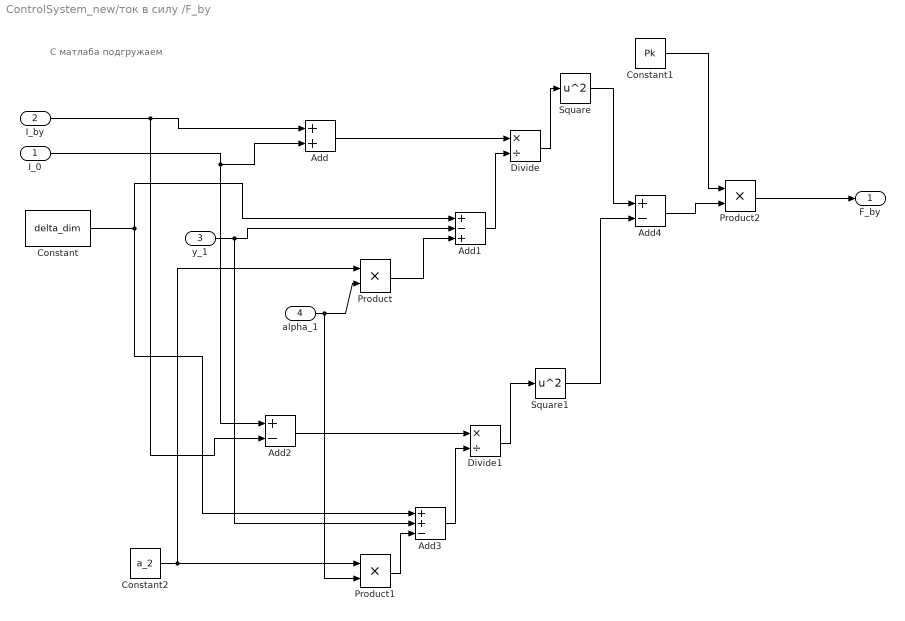
== system ControlSystem_new/ток в силу /F_by ==
  note: С матлаба подгружаем
  I_0 : Inport
  I_by : Inport  Port=2
  y_1 : Inport  Port=3
  alpha_1 : Inport  Port=4
  Add : Sum
  Add1 : Sum  Inputs=+-+
  Add2 : Sum  Inputs=+-
  Add3 : Sum  Inputs=++-
  Add4 : Sum  Inputs=+-
  Constant : Constant  Value=delta_dim
  Constant1 : Constant  Value=Pk
  Constant2 : Constant  Value=a_2
  Divide : Product  Inputs=*/
  Divide1 : Product  Inputs=*/
  Product : Product
  Product1 : Product
  Product2 : Product
  Square : Math  Operator=square  SaturateOnIntegerOverflow=on
  Square1 : Math  Operator=square  SaturateOnIntegerOverflow=on
  F_by : Outport
  wires:
  Product2/1 -> F_by/1
  Constant2/1 -> Product/1, Product1/1
  Product/1 -> Add1/3
  Add1/1 -> Divide/2
  Add/1 -> Divide/1
  Divide/1 -> Square/1
  Product1/1 -> Add3/3
  Add2/1 -> Divide1/1
  I_by/1 -> Add2/2, Add/1
  Add3/1 -> Divide1/2
  y_1/1 -> Add1/2, Add3/2
  Constant/1 -> Add1/1, Add3/1
  Divide1/1 -> Square1/1
  I_0/1 -> Add/2, Add2/1
  alpha_1/1 -> Product/2, Product1/2
  Square/1 -> Add4/1
  Square1/1 -> Add4/2
  Constant1/1 -> Product2/1
  Add4/1 -> Product2/2

== system ControlSystem_new/ток в силу /P ==
  In1 : Inport
  Out1 : Outport
  wires:
  In1/1 -> Out1/1

== system ControlSystem_new/ток в силу /Qv ==
  In1 : Inport
  Out1 : Outport
  wires:
  In1/1 -> Out1/1

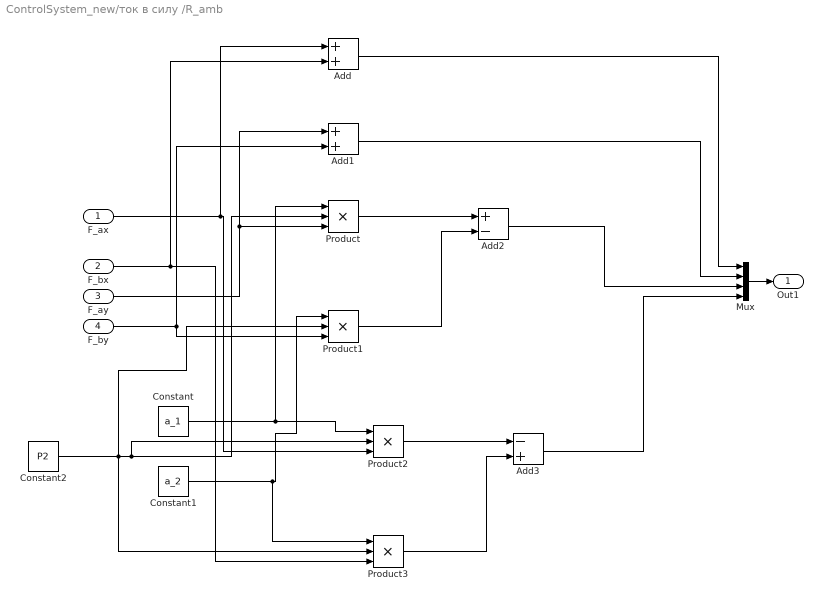
== system ControlSystem_new/ток в силу /R_amb ==
  F_ax : Inport
  F_bx : Inport  Port=2
  F_ay : Inport  Port=3
  F_by : Inport  Port=4
  Add : Sum
  Add1 : Sum
  Add2 : Sum  Inputs=+-
  Add3 : Sum  Inputs=-+
  Constant : Constant  Value=a_1
  Constant1 : Constant  Value=a_2
  Constant2 : Constant  Value=P2
  Mux : Mux
  Product{,1..3} (4 alike) : Product  Inputs=3
  Out1 : Outport
  wires:
  F_ax/1 -> Product2/3, Add/1
  F_bx/1 -> Product3/3, Add/2
  Add/1 -> Mux/1
  F_ay/1 -> Product/3, Add1/1
  F_by/1 -> Product1/3, Add1/2
  Add1/1 -> Mux/2
  Mux/1 -> Out1/1
  Constant/1 -> Product2/1, Product/1
  Product/1 -> Add2/1
  Constant1/1 -> Product3/1, Product1/1
  Product1/1 -> Add2/2
  Add2/1 -> Mux/3
  Product3/1 -> Add3/2
  Product2/1 -> Add3/1
  Add3/1 -> Mux/4
  Constant2/1 -> Product/2, Product2/2, Product3/2, Product1/2

== matlab function ControlSystem_new/Получение момента и силы в виде векторов 1x4 ==
  data: Q_init input; RPM_init input; FMpoints input; Q input; F output; RPM input; M output
function [F,M] = getFM(Q_init,RPM_init,FMpoints,Q,RPM)
% Srfc = struct();
% file = load('Srfc.mat','Srfc');
% Fited = struct();
% Srfc = struct();

% F = zeros(1,4);
% M = zeros(1,4);


f = fit([Q_init, RPM_init],FMpoints,'cubicinterp'); 

figure('Name',"Интерполяция");
title('Интерполяция ');
plot( f, [Q_init, RPM_init],FMpoints)
hold on
xlabel('Q, л/мин')
ylabel('RPM')
zlabel('F/М') 
legend('Эксп.точки')

point_Z = feval(f,Q,RPM);
plot3(Q,RPM,point_Z,"r*",'MarkerSize',10)   
xlabel('Q, л/мин')
ylabel('RPM')
hold off

F=f(Q_to_find,RPM_to_find);
% % m = 1 - Fx, m=2 - Fy, m=3 - Fz, m=4 - Fr, m=5 - Mx и т.д. m=8 - Mr
% for m = 1:8
%     
%     
%     
%      f = Srfc(m).f;
%     
% %     xData = Srfc(m).x;
% %     yData = Srfc(m).y;
% %     zData = Srfc(m).z;
% 
% %     % find point
% %     figure('Name',"Интерполяция");
% %     point_Z = feval(f,Q_to_find,RPM_to_find);
% %     
% %     title('Интерполяция');
% %     plot( f, [xData, yData],zData)
% %     hold on
% %     plot3(Q_to_find,RPM_to_find,point_Z,"r*",'MarkerSize',10)
% %     
% %     xlabel('Q, л/мин')
% %     ylabel('RPM')
% %     if m<=4
% %         zlabel('F, Н')
% %     else
% %         zlabel('М,Н*м')
% %     end
% %     legend('Эксп.точки','Найденное значение', 'Location', 'best', 'Interpreter', 'none' )
% %     hold off
%     
%     % Get Moment or Force values from model
%     if m<5
%         Fited(m).F=f(Q_to_find,RPM_to_find);
%         F(m) = Fitted(m).F; 
%     else
%         Fited(m).M=f(Q_to_find,RPM_to_find);
%         M(m-4) = Fitted(m).M;
%     end
%     
% end
% 

% formatSpec = 'Расход: %4.2f л/мин, частота: %4.0f об/мин\n';
% fprintf(formatSpec,Q,RPM)
% 
% for idx = 1:4
%     if idx == 1
%         name = 'Fx';
%     end
%     if idx == 2
%         name = 'Fy';
%     end
%     if idx == 3
%         name = 'Fz';
%     end
%     if idx == 4
%         name = 'Fr';
%     end
%     formatSpec = 'Сила %s = %4.4f Н\n';
%     fprintf(formatSpec,name,Fited(idx).F);
% end

% F.x = Fited(1).F;
% F.y = Fited(2).F;
% F.z = Fited(3).F;
% F.r = Fited(4).F;
% M.x = Fited(5).M;
% M.y = Fited(6).M;
% M.z = Fited(7).M;
% M.r = Fited(8).M;

end

== matlab function ControlSystem_new/ток в силу /MATLFAB Function ==
  data: u input; y output
function y = fcn(u)

y = u;
